simulink model "model1"  (R2025b)
settings: Solver=VariableStepAuto  StartTime=0.0  StopTime=10.0  RelTol=1e-3
values from neighbouring files (symbols this model uses):
  A = [0 1 0 0 ; 0 -d/m m*g/M 0 ; 0 0 0 1; 0 -d/l*M (M+m)*g/(l*M) 0]    [CartPuller.m]    (also in Controller.m = [0 1 0 0; Ex12_4.m = [-5 1 0;0 -2 1;0 0 -1]; JacobCTP.m = [0 1 0 0; Observer_4state.m = [0 1; -k/m -c/m])
  B = [0 1/M 0 1/(M*l)]'    [CartPuller.m]    (also in Controller.m = [0;1/m1;0;0]; Ex12_4.m = [0;0;1]; Observer_4state.m = [0; 1/m]; full_order_observer_smd.m = [0 0 0 1/m2]')
  C = eye(4)    [Controller.m]    (also in Ex12_4.m = [-1 1 0]; Observer_4state.m = [1 0]; full_order_observer_smd.m = [1 0 0 0]; full_state_observer.m = [1 0 0 0])
  D = zeros(4,1)    [Controller.m]    (also in Ex12_4.m = 0; full_order_observer_smd.m = []; inv_pendulum_lqr.m = m*(L^2)*(M+m*(1-Cx^2)); simulink_observer.m = [])
  K = lqr(A,B,Q,R)    [CartPuller.m]    (also in Ex12_4.m = acker(A,B,poles); full_state_observer.m = place(A', C', poles_o)'; me23b196_asgn4.m = product_of_pole_magnitudes / product_of_zero_magnitudes)
  z0 = [2; 1.5; 1]    [Controller.m]    (also in min_state_observer.m)
undefined symbols (not defined in the file or in its folder): x_ref
settings Model: Creator=Abhi  LastModifiedBy=Abhi

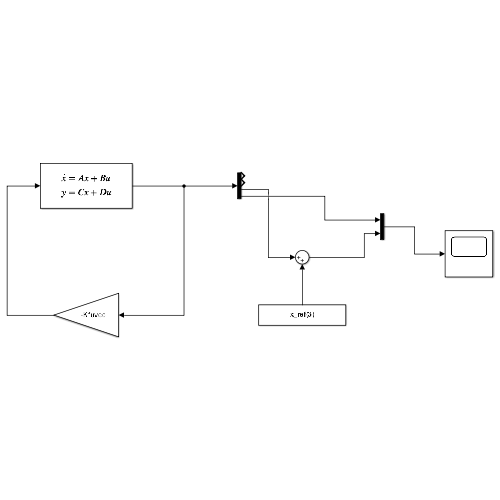
[thumbnail: Simulink's stored preview of the top-level diagram]
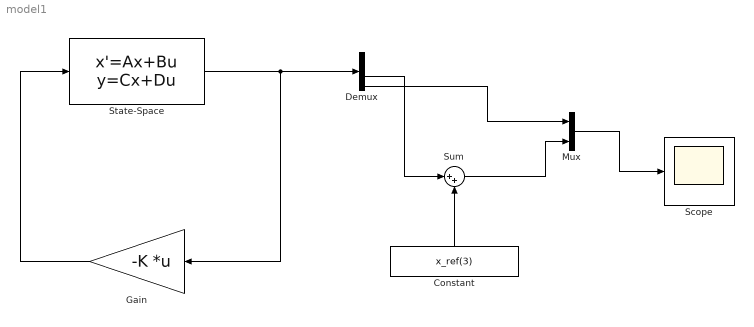
== system model1 ==
  Constant : Constant  Value=x_ref(3)
  Demux : Demux
  Gain : Gain  Gain=-K  Multiplication=Matrix(K*u) (u vector)
  Mux : Mux  Inputs=2
  Scope : Scope
      settings: ActiveDisplayYMinimum=-0.19866768327787895  ActiveDisplayYMaximum=1.7680493505411385
  State-Space : StateSpace  A=A  B=B  C=C  D=D  InitialCondition=z0
  Sum : Sum  Inputs=|++
  wires:
  Gain/1 -> State-Space/1
  State-Space/1 -> Gain/1, Demux/1
  Demux/3 -> Sum/1
  Constant/1 -> Sum/2
  Sum/1 -> Mux/2
  Mux/1 -> Scope/1
  Demux/4 -> Mux/1
